simulink model "EV_PowerLine_AveModel_Simulink_forArch"  (R2023a)
settings: Solver=ode23t  StartTime=0.0  StopTime=2  MaxStep=1e-3  RelTol=1e-3  AbsTol=1e-3
settings Model: PacingRate=1000  Creator=ykamatan  LastModifiedBy=ykamatan
settings SolverCC: AutoScaleAbsTol=off  SolverJacobianMethodControl=SparsePerturbation  DaesscMode=Fast
settings OptimizationCC: ReuseModelBlockBuffer=off
settings DebuggingCC: UnconnectedInputMsg=warning  UnconnectedOutputMsg=warning  UnconnectedLineMsg=warning  SymbolicDimsDataTypeCodeGenerationDiagnostic=none
settings ModelReferenceCC: EnableRefExpFcnMdlSchedulingChecks=on
settings SFSimCC: CustomCodeUndefinedFunction=UseInterfaceOnly
settings RTWCC: DLArmComputeVersion=19.05
settings SimscapeCC: SimscapeLogDataHistory=10000

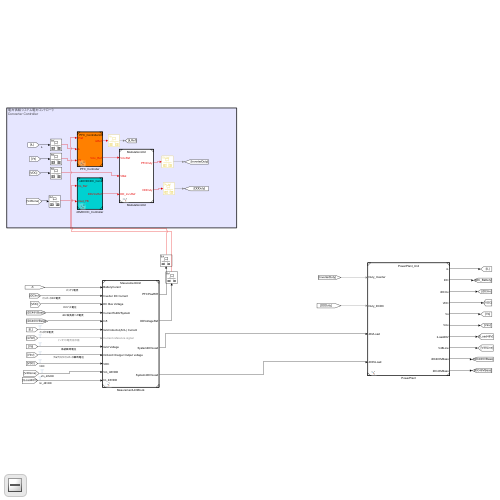
[thumbnail: Simulink's stored preview of the top-level diagram]
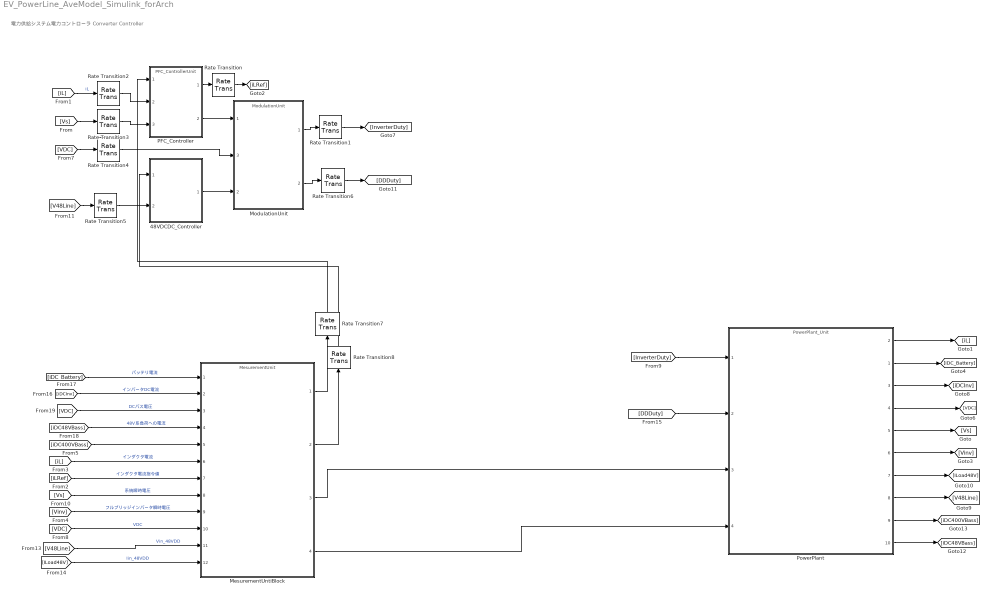
== system EV_PowerLine_AveModel_Simulink_forArch ==
  note: 電力供給システム電力コントローラ
      | Converter Controller
  48VDCDC_Controller : ModelReference  ModelNameDialog=x48VDCDC_Controller_Unit.slx  SimulationMode=Normal  ModelReferenceVersion=5.0
  MesurementUntiBlock : ModelReference  ModelNameDialog=MesurementUnit.slx  SimulationMode=Normal  ModelReferenceVersion=5.0
  ModulationUnit : ModelReference  ModelNameDialog=ModulationUnit  SimulationMode=Normal  ModelReferenceVersion=5.0
      settings: PortSchema="{\"entries\":[{\"content\":{\"sides\":[{\"content\":{\"connectorIds\":[\"In1\",\"In3\",\"In2\"]},\"type\":\"ConnectorPlacement.EquallySpacedRectSide\",\"uuid\":\"118e906f-2ade-41a6-9a4e-068f3bfaf8f6\"},{\"content\":{\"connectorIds\":[\"Out1\",\"Out2\"],\"side\":\"RIGHT\"},\"type\":\"ConnectorPlacement.EquallySpacedRectSide\",\"uuid\":\"d4189a35-2248-4a82-9ac1-3c517fda069d\"},{\"content\":{\"connectorIds\":[],\"side\":\"TOP\"},\"type\":\"ConnectorPlacement.EquallySpacedRectSide\",\"uuid\":\"022377bf-2c76-445c-8b1f-7dbf7ef1f00c\"}]},\"type\":\"ConnectorPlacement.EquallySpacedConnector\",\"uuid\":\"9d61a865-cfcd-4b2d-b31c-7e61bdf759c9\"}],\"packageUris\":[\"http://schema.mathworks.com/mf0/Connector/R2020b\"],\"version\":\"1.0\"}"
  PFC_Controller : ModelReference  ModelNameDialog=PFC_ControllerUnit.slx  SimulationMode=Normal  ModelReferenceVersion=5.0
  PowerPlant : ModelReference  ModelNameDialog=PowerPlant_Unit.slx  SimulationMode=Normal  ModelReferenceVersion=5.0
      settings: PortSchema="{\"entries\":[{\"content\":{\"sides\":[{\"content\":{\"connectorIds\":[\"In1\",\"In2\",\"In3\",\"In4\"]},\"type\":\"ConnectorPlacement.EquallySpacedRectSide\",\"uuid\":\"d29d321e-d4c1-4367-9f49-8ab499eecf0c\"},{\"content\":{\"connectorIds\":[\"Out2\",\"Out1\",\"Out3\",\"Out4\",\"Out5\",\"Out6\",\"Out7\",\"Out8\",\"Out9\",\"Out10\"],\"side\":\"RIGHT\"},\"type\":\"ConnectorPlacement.EquallySpacedRectSide\",\"uuid\":\"4d8fa41c-fb31-4713-93b3-c48cd1c08f8c\"},{\"content\":{\"connectorIds\":[],\"side\":\"TOP\"},\"type\":\"ConnectorPlacement.EquallySpacedRectSide\",\"uuid\":\"adfa6be3-4dbd-435f-869f-803a17683fc1\"}]},\"type\":\"ConnectorPlacement.EquallySpacedConnector\",\"uuid\":\"1988591c-f17a-4348-a64a-e9a0ebcd7430\"}],\"packageUris\":[\"http://schema.mathworks.com/mf0/Connector/R2020b\"],\"version\":\"1.0\"}"
  Rate Transition : RateTransition
  Rate Transition{1..8} (8 alike) : RateTransition  Deterministic=off
  wires:
  [iL] -> Rate Transition2/1  "iL"
  PFC_Controller/1 -> Rate Transition/1
  PFC_Controller/2 -> ModulationUnit/1
  MesurementUntiBlock/2 -> Rate Transition8/1
  48VDCDC_Controller/1 -> ModulationUnit/2
  [InverterDuty] -> PowerPlant/1
  [DDDuty] -> PowerPlant/2
  PowerPlant/1 -> [iDC_Battery]
  PowerPlant/2 -> [iL]
  [V48Line] -> Rate Transition5/1
  [VDC] -> Rate Transition4/1
  [Vs] -> Rate Transition3/1
  Rate Transition5/1 -> 48VDCDC_Controller/2
  Rate Transition4/1 -> ModulationUnit/3
  Rate Transition/1 -> [iLRef]
  Rate Transition1/1 -> [InverterDuty]
  Rate Transition6/1 -> [DDDuty]
  PowerPlant/3 -> [iDCInv]
  PowerPlant/4 -> [VDC]
  PowerPlant/5 -> [Vs]
  PowerPlant/6 -> [Vinv]
  PowerPlant/7 -> [ILoad48V]
  PowerPlant/8 -> [V48Line]
  PowerPlant/9 -> [iDC400VBass]
  PowerPlant/10 -> [iDC48VBass]
  ModulationUnit/1 -> Rate Transition1/1
  ModulationUnit/2 -> Rate Transition6/1
  MesurementUntiBlock/1 -> Rate Transition7/1
  [iDC_Battery] -> MesurementUntiBlock/1  "バッテリ電流"
  [iDCInv] -> MesurementUntiBlock/2  "インバータDC電流"
  [VDC] -> MesurementUntiBlock/3  "DCバス電圧"
  [iDC48VBass] -> MesurementUntiBlock/4  "48V系負荷への電流"
  [iDC400VBass] -> MesurementUntiBlock/5
  [iL] -> MesurementUntiBlock/6  "インダクタ電流"
  [iLRef] -> MesurementUntiBlock/7  "インダクタ電流指令値"
  [Vs] -> MesurementUntiBlock/8  "系統瞬時電圧"
  [Vinv] -> MesurementUntiBlock/9  "フルブリッジインバータ瞬時電圧"
  [VDC] -> MesurementUntiBlock/10  "VDC"
  [V48Line] -> MesurementUntiBlock/11  "Vin_48VDD"
  [ILoad48V] -> MesurementUntiBlock/12  "Iin_48VDD"
  MesurementUntiBlock/3 -> PowerPlant/3
  Rate Transition2/1 -> PFC_Controller/2
  Rate Transition3/1 -> PFC_Controller/3
  MesurementUntiBlock/4 -> PowerPlant/4
  Rate Transition7/1 -> PFC_Controller/1
  Rate Transition8/1 -> 48VDCDC_Controller/1
